simulink model "Mode0"  (R2023b)
settings: Solver=VariableStepAuto  StartTime=0.0  StopTime=10.0  RelTol=1e-3
values from neighbouring files (symbols this model uses):
  w_c_val = 0.05    [phase_portrait.m]
undefined symbols (not defined in the file or in its folder): deadband, I1, I2, I3, Is, K_d, K_p, td, thd_0, tmax
settings Model: Creator=Connor Emmons  LastModifiedBy=Connor Emmons

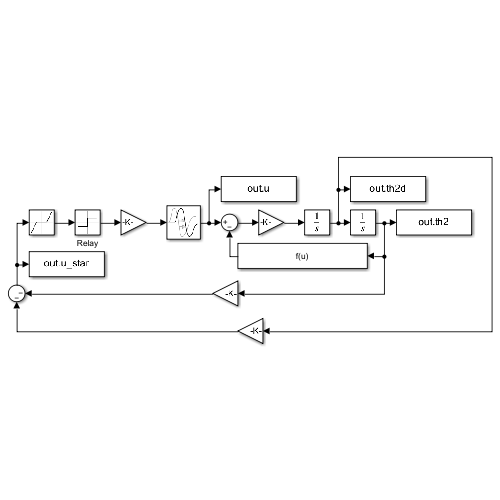
[thumbnail: Simulink's stored preview of the top-level diagram]
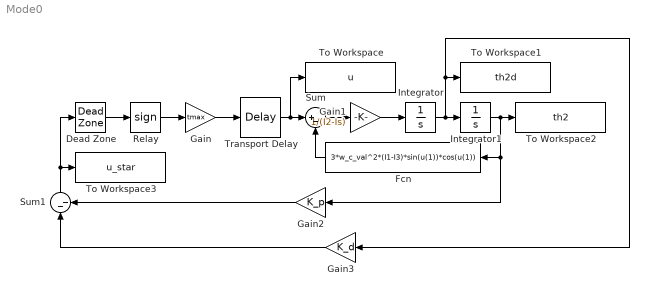
== system Mode0 ==
  Dead Zone : DeadZone  LowerValue=-deadband  UpperValue=deadband
  Fcn : Fcn  Expr=3*w_c_val^2*(I1-I3)*sin(u(1))*cos(u(1))
  Gain : Gain  Gain=tmax
  Gain1 : Gain  Gain=1/(I2-Is)
  Gain2 : Gain  Gain=K_p
  Gain3 : Gain  Gain=K_d
  Integrator : Integrator  InitialCondition=thd_0
  Integrator1 : Integrator
  Relay : Signum
  Sum : Sum  Inputs=|+-
  Sum1 : Sum  Inputs=|--
  To Workspace : ToWorkspace  VariableName=u  SampleTime=-1
  To Workspace1 : ToWorkspace  VariableName=th2d  SampleTime=-1
  To Workspace2 : ToWorkspace  VariableName=th2  SampleTime=-1
  To Workspace3 : ToWorkspace  VariableName=u_star  SampleTime=-1
  Transport Delay : TransportDelay  DelayTime=td
  wires:
  Relay/1 -> Gain/1
  Gain/1 -> Transport Delay/1
  Transport Delay/1 -> To Workspace/1, Sum/1
  Sum/1 -> Gain1/1
  Gain1/1 -> Integrator/1
  Integrator/1 -> Gain3/1, To Workspace1/1, Integrator1/1
  Integrator1/1 -> Gain2/1, Fcn/1, To Workspace2/1
  Fcn/1 -> Sum/2
  Dead Zone/1 -> Relay/1
  Sum1/1 -> Dead Zone/1, To Workspace3/1
  Gain2/1 -> Sum1/2
  Gain3/1 -> Sum1/1
